simulink model "six_dof_mock"  (Simulink 7.1)
settings: Solver=ode45  StartTime=0.0  StopTime=30  MaxStep=.01  RelTol=1e-3
libraries: simulink x3, aero_sim_lib x1
settings Model: Creator=Administrator  LastModifiedBy=Administrator

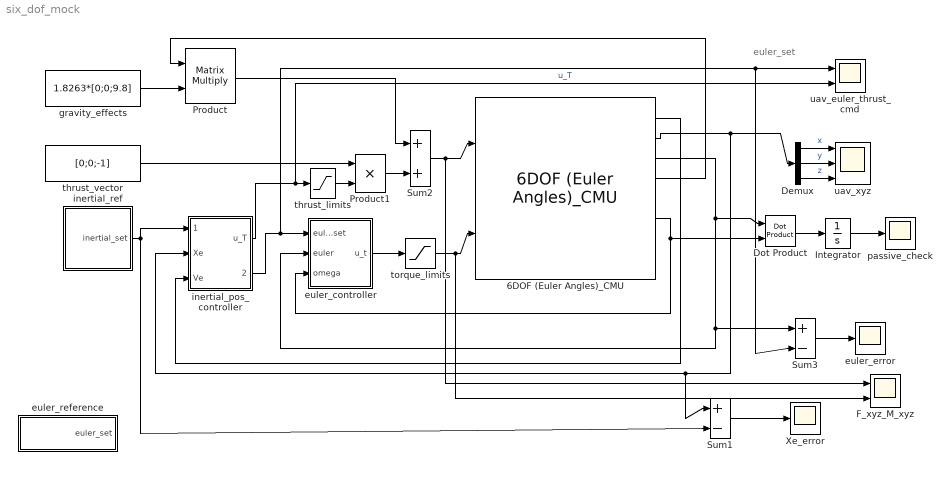
== system six_dof_mock ==
  note: euler_set
  6DOF (Euler Angles)_CMU : aero_sim_lib/6DOF (Euler Angles)_CMU  SystemSampleTime=-1  XYZe_0=zeros(3,1)  Vb_0=zeros(3,1)  euler_0=zeros(3,1)  omega_0=zeros(3,1)  M=1.8263  I=diag([0.02759 0.02771 0.04806])
  Demux : Demux  Outputs=[1 1 1]
  Dot Product : simulink/Math Operations/Dot Product  InputSameDT=on  OutDataType=sfix(16)  OutScaling=2^-10  DoSatur=off
  F_xyz_M_xyz : Scope  NumInputPorts=2
      settings: YMin=-1.047197551196598~10  YMax=1.047197551196598~30  SaveName=ScopeData5
  Integrator : Integrator
  Product : Product  Multiplication=Matrix(*)  OutDataType=sfix(16)  OutScaling=2^0  RndMeth=Zero
  Product1 : Product  OutDataType=sfix(16)  OutScaling=2^0  RndMeth=Zero
  Sum1 : Sum  Inputs=|+-  OutDataType=sfix(16)  OutScaling=2^0
  Sum2 : Sum  Inputs=|++  OutDataType=sfix(16)  OutScaling=2^0
  Sum3 : Sum  Inputs=|+-  OutDataType=sfix(16)  OutScaling=2^0
  Xe_error : Scope
      settings: YMin=-4  YMax=4  SaveName=ScopeData3
  euler_controller : Subsystem  mask{K=25, K_v=1}
  euler_error : Scope
      settings: YMin=-4  YMax=4  SaveName=ScopeData4
  euler_reference : Subsystem
  gravity_effects : Constant  Value=1.8263*[0;0;9.8]  OutDataType=sfix(16)  OutScaling=2^0
  inertial_pos_controller : Subsystem  mask{Ts=.01, M=1.8263, K=10, K_Ve=4}
      mask prompts: Ts "Enter Sample Time [Ts] (seconds):"; M "Enter Mass of UAV [M] (kg):"; K "Enter Loop Gain [K]:"; K_Ve "Enter Velocity Damping Gain [K_Ve]:"
  inertial_ref : Subsystem
  passive_check : Scope
      settings: YMin=-22500  YMax=2500  SaveName=ScopeData2
  thrust_limits : Saturate  UpperLimit=9.8*4  LowerLimit=0  OutDataType=sfix(16)  OutScaling=2^0
  thrust_vector : Constant  Value=[0;0;-1]  OutDataType=sfix(16)  OutScaling=2^0
  torque_limits : Saturate  UpperLimit=12*ones(3,1)  LowerLimit=-12*ones(3,1)  OutDataType=sfix(16)  OutScaling=2^0
  uav_euler_thrust_cmd : Scope  NumInputPorts=2
      settings: YMin=-1.047197551196598~10  YMax=1.047197551196598~30
  uav_xyz : Scope  NumInputPorts=3
      settings: YMin=-22500~-5~-5  YMax=2500~5~5
  wires:
  6DOF (Euler Angles)_CMU/3 -> Dot Product/1, euler_controller/2(euler), Sum3/1
  torque_limits/1 -> 6DOF (Euler Angles)_CMU/2, F_xyz_M_xyz/2
  euler_controller/1(u_t) -> torque_limits/1
  gravity_effects/1 -> Product/2
  6DOF (Euler Angles)_CMU/4 -> Product/1
  Product/1 -> Sum2/1
  thrust_vector/1 -> Product1/1
  Dot Product/1 -> Integrator/1
  Integrator/1 -> passive_check/1
  Sum2/1 -> 6DOF (Euler Angles)_CMU/1, F_xyz_M_xyz/1
  inertial_pos_controller/1(u_T) -> uav_euler_thrust_cmd/2, thrust_limits/1  "u_T"
  inertial_pos_controller/2(u_euler) -> euler_controller/1(euler_set), uav_euler_thrust_cmd/1, Sum3/2
  Product1/1 -> Sum2/2
  inertial_ref/1(inertial_set) -> inertial_pos_controller/1(Xe_set), Sum1/2
  6DOF (Euler Angles)_CMU/2 -> Demux/1, inertial_pos_controller/2(Xe), Sum1/1
  Demux/1 -> uav_xyz/1  "x"
  Demux/2 -> uav_xyz/2  "y"
  Demux/3 -> uav_xyz/3  "z"
  6DOF (Euler Angles)_CMU/1 -> inertial_pos_controller/3(Ve)
  thrust_limits/1 -> Product1/2
  6DOF (Euler Angles)_CMU/6 -> Dot Product/2, euler_controller/3(omega)
  Sum1/1 -> Xe_error/1
  Sum3/1 -> euler_error/1

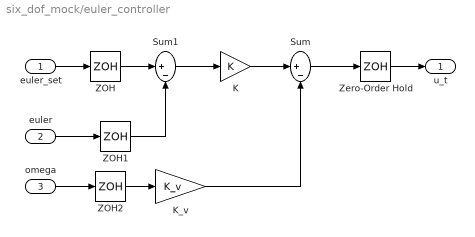
== system six_dof_mock/euler_controller ==
  euler_set : Inport
  euler : Inport  Port=2
  omega : Inport  Port=3
  K : Gain  Gain=K  ParameterDataType=sfix(16)  ParameterScaling=2^0  OutDataType=sfix(16)  OutScaling=2^0
  K_v : Gain  Gain=K_v  ParameterDataType=sfix(16)  ParameterScaling=2^0  OutDataType=sfix(16)  OutScaling=2^0
  Sum : Sum  Inputs=|+-  OutDataType=sfix(16)  OutScaling=2^0
  Sum1 : Sum  Inputs=|+-  OutDataType=sfix(16)  OutScaling=2^0
  ZOH : ZeroOrderHold  SampleTime=.01
  ZOH1 : ZeroOrderHold  SampleTime=.01
  ZOH2 : ZeroOrderHold  SampleTime=.01
  Zero-Order Hold : ZeroOrderHold  SampleTime=.01
  u_t : Outport
  wires:
  Sum/1 -> Zero-Order Hold/1
  K_v/1 -> Sum/2
  ZOH2/1 -> K_v/1
  euler/1 -> ZOH1/1
  euler_set/1 -> ZOH/1
  Zero-Order Hold/1 -> u_t/1
  omega/1 -> ZOH2/1
  K/1 -> Sum/1
  ZOH/1 -> Sum1/1
  Sum1/1 -> K/1
  ZOH1/1 -> Sum1/2

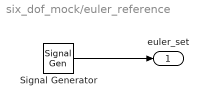
== system six_dof_mock/euler_reference ==
  Signal Generator : SignalGenerator  WaveForm=square  Amplitude=(pi*.75*58/180)*[1 -1 0]  Frequency=.25*ones(3,1)
  euler_set : Outport
  wires:
  Signal Generator/1 -> euler_set/1

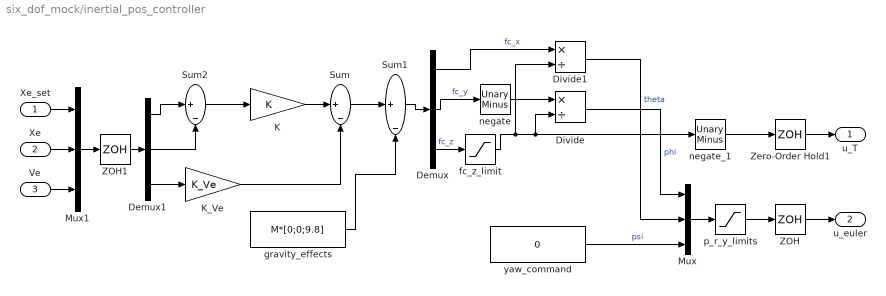
== system six_dof_mock/inertial_pos_controller ==
  Xe_set : Inport
  Xe : Inport  Port=2
  Ve : Inport  Port=3
  Demux : Demux  Outputs=[1 1 1]
  Demux1 : Demux  Outputs=[3 3 3]
  Divide : Product  Inputs=*/  OutDataType=sfix(16)  OutScaling=2^-10
  Divide1 : Product  Inputs=*/  OutDataType=sfix(16)  OutScaling=2^-10
  K : Gain  Gain=K  ParameterDataType=sfix(16)  ParameterScaling=2^0  OutDataType=sfix(16)  OutScaling=2^0
  K_Ve : Gain  Gain=K_Ve  ParameterDataType=sfix(16)  ParameterScaling=2^0  OutDataType=sfix(16)  OutScaling=2^0
  Mux : Mux  Inputs=[1 1 1]
  Mux1 : Mux  Inputs=[3 3 3]
  Sum : Sum  Inputs=|+-  OutDataType=sfix(16)  OutScaling=2^0
  Sum1 : Sum  Inputs=|+-  OutDataType=sfix(16)  OutScaling=2^0
  Sum2 : Sum  Inputs=|+-  OutDataType=sfix(16)  OutScaling=2^0
  ZOH : ZeroOrderHold  SampleTime=Ts
  ZOH1 : ZeroOrderHold  SampleTime=Ts
  Zero-Order Hold1 : ZeroOrderHold  SampleTime=Ts
  fc_z_limit : Saturate  UpperLimit=-(1/4)*9.81  LowerLimit=-4*9.81  OutDataType=sfix(16)  OutScaling=2^0
  gravity_effects : Constant  Value=M*[0;0;9.8]  OutDataType=sfix(16)  OutScaling=2^0
  negate : simulink/Math Operations/Unary Minus  DoSatur=off
  negate_1 : simulink/Math Operations/Unary Minus  DoSatur=off
  p_r_y_limits : Saturate  UpperLimit=(pi/4)*ones(3,1)  LowerLimit=-(pi/4)*ones(3,1)  OutDataType=sfix(16)  OutScaling=2^0
  yaw_command : Constant  Value=0  OutDataType=sfix(16)  OutScaling=2^0
  u_T : Outport
  u_euler : Outport  Port=2
  wires:
  ZOH/1 -> u_euler/1
  gravity_effects/1 -> Sum1/2
  Zero-Order Hold1/1 -> u_T/1
  Sum1/1 -> Demux/1
  Mux/1 -> p_r_y_limits/1
  Demux/3 -> fc_z_limit/1  "fc_z"
  yaw_command/1 -> Mux/3  "psi"
  Demux/2 -> negate/1  "fc_y"
  negate/1 -> Divide/1
  Divide/1 -> Mux/1  "phi"
  Demux/1 -> Divide1/1  "fc_x"
  Divide1/1 -> Mux/2  "theta"
  p_r_y_limits/1 -> ZOH/1
  negate_1/1 -> Zero-Order Hold1/1
  Xe_set/1 -> Mux1/1
  Xe/1 -> Mux1/2
  Ve/1 -> Mux1/3
  Mux1/1 -> ZOH1/1
  ZOH1/1 -> Demux1/1
  Demux1/3 -> K_Ve/1
  fc_z_limit/1 -> Divide/2, negate_1/1, Divide1/2
  K/1 -> Sum/1
  K_Ve/1 -> Sum/2
  Sum/1 -> Sum1/1
  Sum2/1 -> K/1
  Demux1/1 -> Sum2/1
  Demux1/2 -> Sum2/2

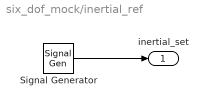
== system six_dof_mock/inertial_ref ==
  Signal Generator : SignalGenerator  Amplitude=10*[1 -1 1]  Frequency=.0625*ones(3,1)
  inertial_set : Outport
  wires:
  Signal Generator/1 -> inertial_set/1
